simulink model "dinamica_pata_simulink"  (R2023b)
settings: Solver=ode45  StartTime=0.0  StopTime=2.5  MaxStep=0.001  RelTol=1e-9  AbsTol=1e-11
values from neighbouring files (symbols this model uses):
  sim_pata = struct('theta0', E.theta0, 'dtheta0', E.dtheta0,      't_final', E.t_final)    [INICIAR_DINAMICA_PATA.m]    (also in analizar_energia_solver.m = struct('theta0', theta0, 'dtheta0', dtheta0,      't_final',; simular_dinamica_pata.m = struct('theta0', E.theta0, 'dtheta0', E.dtheta0, 't_final', )
undefined symbols (not defined in the file or in its folder): par_pata
libraries: simulink x6
settings Model: Creator=matia  LastModifiedBy=matia

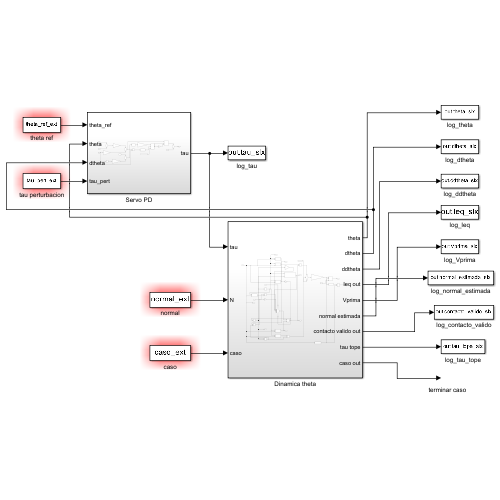
[thumbnail: Simulink's stored preview of the top-level diagram]
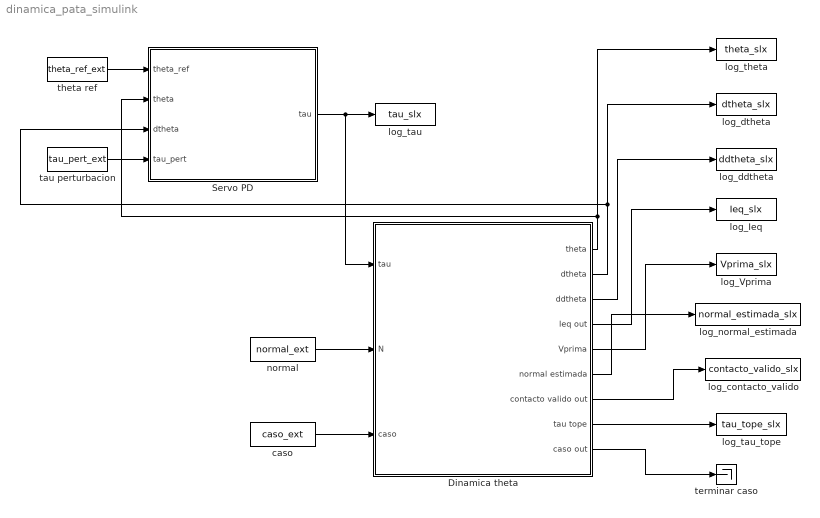
== system dinamica_pata_simulink ==
  Dinamica theta : Subsystem
  Servo PD : Subsystem
  caso : FromWorkspace  VariableName=caso_ext  OutputAfterFinalValue=Holding final value
  log_Ieq : ToWorkspace  VariableName=Ieq_slx  SaveFormat=Timeseries  SampleTime=-1
  log_Vprima : ToWorkspace  VariableName=Vprima_slx  SaveFormat=Timeseries  SampleTime=-1
  log_contacto_valido : ToWorkspace  VariableName=contacto_valido_slx  SaveFormat=Timeseries  SampleTime=-1
  log_ddtheta : ToWorkspace  VariableName=ddtheta_slx  SaveFormat=Timeseries  SampleTime=-1
  log_dtheta : ToWorkspace  VariableName=dtheta_slx  SaveFormat=Timeseries  SampleTime=-1
  log_normal_estimada : ToWorkspace  VariableName=normal_estimada_slx  SaveFormat=Timeseries  SampleTime=-1
  log_tau : ToWorkspace  VariableName=tau_slx  SaveFormat=Timeseries  SampleTime=-1
  log_tau_tope : ToWorkspace  VariableName=tau_tope_slx  SaveFormat=Timeseries  SampleTime=-1
  log_theta : ToWorkspace  VariableName=theta_slx  SaveFormat=Timeseries  SampleTime=-1
  normal : FromWorkspace  VariableName=normal_ext  OutputAfterFinalValue=Holding final value
  tau perturbacion : FromWorkspace  VariableName=tau_pert_ext  OutputAfterFinalValue=Holding final value
  terminar caso : Terminator
  theta ref : FromWorkspace  VariableName=theta_ref_ext  OutputAfterFinalValue=Holding final value
  wires:
  Dinamica theta/7(contacto valido out) -> log_contacto_valido/1
  theta ref/1 -> Servo PD/1(theta_ref)
  normal/1 -> Dinamica theta/2(N)
  Dinamica theta/3(ddtheta) -> log_ddtheta/1
  Dinamica theta/6(normal estimada) -> log_normal_estimada/1
  Dinamica theta/2(dtheta) -> Servo PD/3(dtheta), log_dtheta/1
  Dinamica theta/1(theta) -> Servo PD/2(theta), log_theta/1
  Dinamica theta/8(tau tope) -> log_tau_tope/1
  Dinamica theta/5(Vprima) -> log_Vprima/1
  caso/1 -> Dinamica theta/3(caso)
  Servo PD/1(tau) -> Dinamica theta/1(tau), log_tau/1
  tau perturbacion/1 -> Servo PD/4(tau_pert)
  Dinamica theta/9(caso out) -> terminar caso/1
  Dinamica theta/4(Ieq out) -> log_Ieq/1

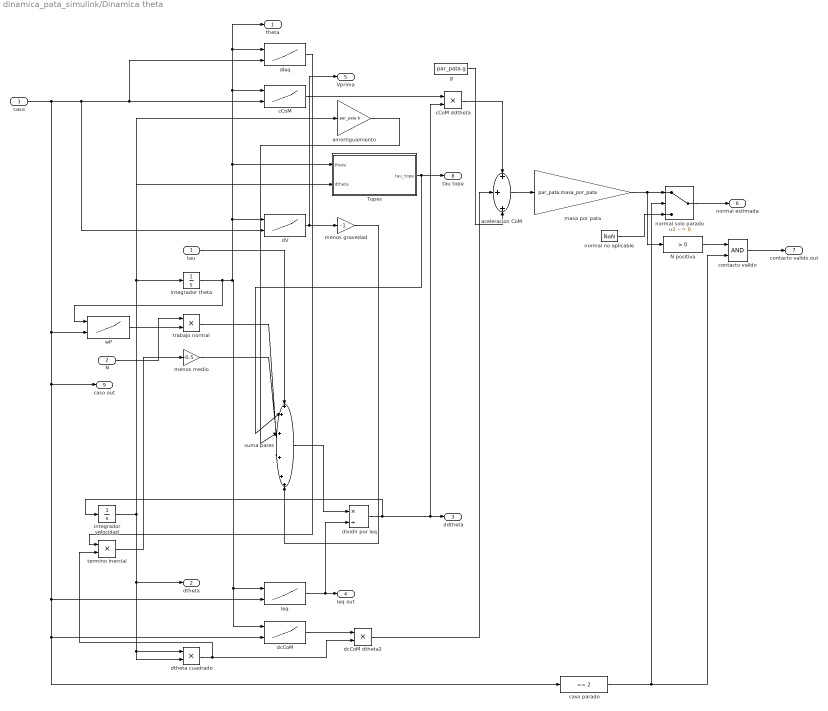
== system dinamica_pata_simulink/Dinamica theta ==
  tau : Inport
  N : Inport  Port=2
  caso : Inport  Port=3
  Ieq : Lookup_n-D  BreakpointsForDimension1=par_pata.theta  BreakpointsForDimension2=par_pata.casos  BreakpointsForDimension3=[5, 7]  Table=par_pata.Ieq  ExtrapMethod=Clip  InternalRulePriority=Speed  RndMeth=Simplest
      settings: InputPortMap=u0,u1
  N positiva : simulink/Logic and Bit Operations/Compare To Zero  relop=>  OutDataTypeStr=boolean
  Topes : Subsystem
  aceleracion CoM : Sum  Inputs=+++
  amortiguamiento : Gain  Gain=-par_pata.b
  cCoM : Lookup_n-D  BreakpointsForDimension1=par_pata.theta  BreakpointsForDimension2=par_pata.casos  BreakpointsForDimension3=[5, 7]  Table=par_pata.cCoM  ExtrapMethod=Clip  InternalRulePriority=Speed  RndMeth=Simplest
      settings: InputPortMap=u0,u1
  cCoM ddtheta : Product  Inputs=**
  caso parado : simulink/Logic and Bit Operations/Compare To Constant  relop===  const=2  OutDataTypeStr=boolean
  contacto valido : Logic  AllPortsSameDT=off  OutDataTypeStr=boolean
  dIeq : Lookup_n-D  BreakpointsForDimension1=par_pata.theta  BreakpointsForDimension2=par_pata.casos  BreakpointsForDimension3=[5, 7]  Table=par_pata.dIeq  ExtrapMethod=Clip  InternalRulePriority=Speed  RndMeth=Simplest
      settings: InputPortMap=u0,u1
  dV : Lookup_n-D  BreakpointsForDimension1=par_pata.theta  BreakpointsForDimension2=par_pata.casos  BreakpointsForDimension3=[5, 7]  Table=par_pata.dV  ExtrapMethod=Clip  InternalRulePriority=Speed  RndMeth=Simplest
      settings: InputPortMap=u0,u1
  dcCoM : Lookup_n-D  BreakpointsForDimension1=par_pata.theta  BreakpointsForDimension2=par_pata.casos  BreakpointsForDimension3=[5, 7]  Table=par_pata.dcCoM  ExtrapMethod=Clip  InternalRulePriority=Speed  RndMeth=Simplest
      settings: InputPortMap=u0,u1
  dcCoM dtheta2 : Product  Inputs=**
  dividir por Ieq : Product  Inputs=*/
  dtheta cuadrado : Product  Inputs=**
  g : Constant  Value=par_pata.g
  integrador theta : Integrator  InitialCondition=sim_pata.theta0
  integrador velocidad : Integrator  InitialCondition=sim_pata.dtheta0
  masa por pata : Gain  Gain=par_pata.masa_por_pata
  menos gravedad : Gain  Gain=-1
  menos medio : Gain  Gain=-0.5
  normal no aplicable : Constant  Value=NaN
  normal solo parado : Switch  Criteria=u2 ~= 0  SaturateOnIntegerOverflow=off  InputSameDT=off
  suma pares : Sum  Inputs=++++++
  termino inercial : Product  Inputs=**
  trabajo normal : Product  Inputs=**
  wP : Lookup_n-D  BreakpointsForDimension1=par_pata.theta  BreakpointsForDimension2=par_pata.casos  BreakpointsForDimension3=[5, 7]  Table=par_pata.wP  ExtrapMethod=Clip  InternalRulePriority=Speed  RndMeth=Simplest
      settings: InputPortMap=u0,u1
  theta : Outport
  dtheta : Outport  Port=2
  ddtheta : Outport  Port=3
  Ieq out : Outport  Port=4
  Vprima : Outport  Port=5
  normal estimada : Outport  Port=6
  contacto valido out : Outport  Port=7
  tau tope : Outport  Port=8
  caso out : Outport  Port=9
  wires:
  tau/1 -> suma pares/1
  N/1 -> trabajo normal/1
  N positiva/1 -> contacto valido/1
  caso/1 -> caso parado/1, dcCoM/2, Ieq/2, caso out/1, wP/2, cCoM/2, dIeq/2, dV/2
  trabajo normal/1 -> suma pares/4
  termino inercial/1 -> menos medio/1
  wP/1 -> trabajo normal/2
  menos medio/1 -> suma pares/5
  integrador velocidad/1 -> dtheta cuadrado/2, dtheta cuadrado/1, dtheta/1, amortiguamiento/1, integrador theta/1, Topes/2(dtheta)
  dcCoM dtheta2/1 -> aceleracion CoM/2
  integrador theta/1 -> dcCoM/1, Ieq/1, dIeq/1, theta/1, cCoM/1, Topes/1(theta), dV/1, wP/1
  dIeq/1 -> termino inercial/1
  dtheta cuadrado/1 -> termino inercial/2, dcCoM dtheta2/2
  cCoM/1 -> cCoM ddtheta/1
  dividir por Ieq/1 -> cCoM ddtheta/2, ddtheta/1, integrador velocidad/1
  dcCoM/1 -> dcCoM dtheta2/1
  dV/1 -> menos gravedad/1, Vprima/1
  suma pares/1 -> dividir por Ieq/1
  Ieq/1 -> dividir por Ieq/2, Ieq out/1
  amortiguamiento/1 -> suma pares/3
  Topes/1(tau_tope) -> tau tope/1, suma pares/2
  normal solo parado/1 -> normal estimada/1
  normal no aplicable/1 -> normal solo parado/3
  menos gravedad/1 -> suma pares/6
  g/1 -> aceleracion CoM/3
  cCoM ddtheta/1 -> aceleracion CoM/1
  aceleracion CoM/1 -> masa por pata/1
  masa por pata/1 -> N positiva/1, normal solo parado/1
  contacto valido/1 -> contacto valido out/1
  caso parado/1 -> contacto valido/2, normal solo parado/2

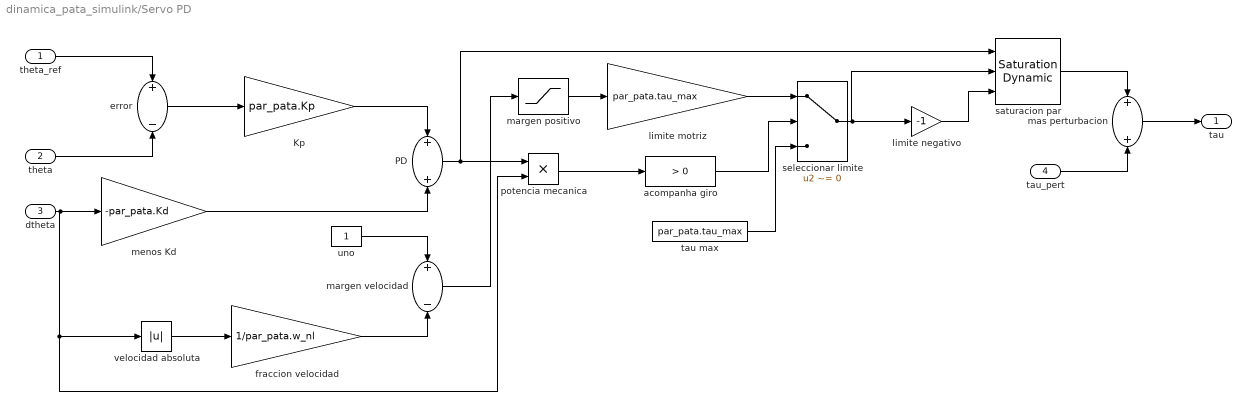
== system dinamica_pata_simulink/Servo PD ==
  theta_ref : Inport
  theta : Inport  Port=2
  dtheta : Inport  Port=3
  tau_pert : Inport  Port=4
  Kp : Gain  Gain=par_pata.Kp
  PD : Sum
  acompanha giro : simulink/Logic and Bit Operations/Compare To Zero  relop=>  OutDataTypeStr=boolean
  error : Sum  Inputs=+-
  fraccion velocidad : Gain  Gain=1/par_pata.w_nl
  limite motriz : Gain  Gain=par_pata.tau_max
  limite negativo : Gain  Gain=-1
  margen positivo : Saturate  UpperLimit=1  LowerLimit=0
  margen velocidad : Sum  Inputs=+-
  mas perturbacion : Sum
  menos Kd : Gain  Gain=-par_pata.Kd
  potencia mecanica : Product  Inputs=**
  saturacion par : simulink/Discontinuities/Saturation Dynamic  OutMin=[]  OutMax=[]  OutDataTypeStr=Inherit: Same as second input  OutDataType=fixdt(1, 16)  OutScaling=2^-10  DoSatur=off
  seleccionar limite : Switch  Criteria=u2 ~= 0  SaturateOnIntegerOverflow=off  InputSameDT=off
  tau max : Constant  Value=par_pata.tau_max
  uno : Constant
  velocidad absoluta : Abs  SaturateOnIntegerOverflow=off
  tau : Outport
  wires:
  dtheta/1 -> potencia mecanica/2, velocidad absoluta/1, menos Kd/1
  theta/1 -> error/2
  theta_ref/1 -> error/1
  Kp/1 -> PD/1
  margen positivo/1 -> limite motriz/1
  error/1 -> Kp/1
  PD/1 -> saturacion par/1, potencia mecanica/1
  menos Kd/1 -> PD/2
  uno/1 -> margen velocidad/1
  velocidad absoluta/1 -> fraccion velocidad/1
  fraccion velocidad/1 -> margen velocidad/2
  margen velocidad/1 -> margen positivo/1
  seleccionar limite/1 -> saturacion par/2, limite negativo/1
  potencia mecanica/1 -> acompanha giro/1
  limite motriz/1 -> seleccionar limite/1
  tau_pert/1 -> mas perturbacion/2
  acompanha giro/1 -> seleccionar limite/2
  saturacion par/1 -> mas perturbacion/1
  tau max/1 -> seleccionar limite/3
  limite negativo/1 -> saturacion par/3
  mas perturbacion/1 -> tau/1

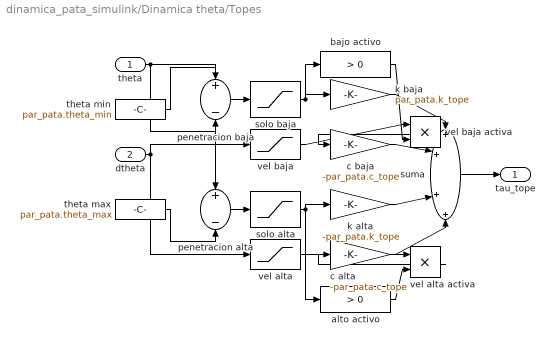
== system dinamica_pata_simulink/Dinamica theta/Topes ==
  theta : Inport
  dtheta : Inport  Port=2
  alto activo : simulink/Logic and Bit Operations/Compare To Zero  relop=>  OutDataTypeStr=boolean
  bajo activo : simulink/Logic and Bit Operations/Compare To Zero  relop=>  OutDataTypeStr=boolean
  c alta : Gain  Gain=-par_pata.c_tope
  c baja : Gain  Gain=-par_pata.c_tope
  k alta : Gain  Gain=-par_pata.k_tope
  k baja : Gain  Gain=par_pata.k_tope
  penetracion alta : Sum  Inputs=+-
  penetracion baja : Sum  Inputs=+-
  solo alta : Saturate  UpperLimit=inf  LowerLimit=0
  solo baja : Saturate  UpperLimit=inf  LowerLimit=0
  suma : Sum  Inputs=++++
  theta max : Constant  Value=par_pata.theta_max
  theta min : Constant  Value=par_pata.theta_min
  vel alta : Saturate  UpperLimit=inf  LowerLimit=0
  vel alta activa : Product  Inputs=**
  vel baja : Saturate  UpperLimit=0  LowerLimit=-inf
  vel baja activa : Product  Inputs=**
  tau_tope : Outport
  wires:
  theta min/1 -> penetracion baja/1
  theta/1 -> penetracion baja/2, penetracion alta/1
  theta max/1 -> penetracion alta/2
  penetracion baja/1 -> solo baja/1
  penetracion alta/1 -> solo alta/1
  dtheta/1 -> vel baja/1, vel alta/1
  solo baja/1 -> k baja/1, bajo activo/1
  solo alta/1 -> k alta/1, alto activo/1
  vel baja/1 -> vel baja activa/1
  bajo activo/1 -> vel baja activa/2
  vel alta/1 -> vel alta activa/1
  alto activo/1 -> vel alta activa/2
  vel baja activa/1 -> c baja/1
  vel alta activa/1 -> c alta/1
  k baja/1 -> suma/1
  c baja/1 -> suma/2
  k alta/1 -> suma/3
  c alta/1 -> suma/4
  suma/1 -> tau_tope/1
